simulink model "mds_3c"  (R2014a)
settings: Solver=ode3  StartTime=0.0  StopTime=120  FixedStep=0.002  RelTol=1e-3
settings Model: Creator=john  LastModifiedBy=john

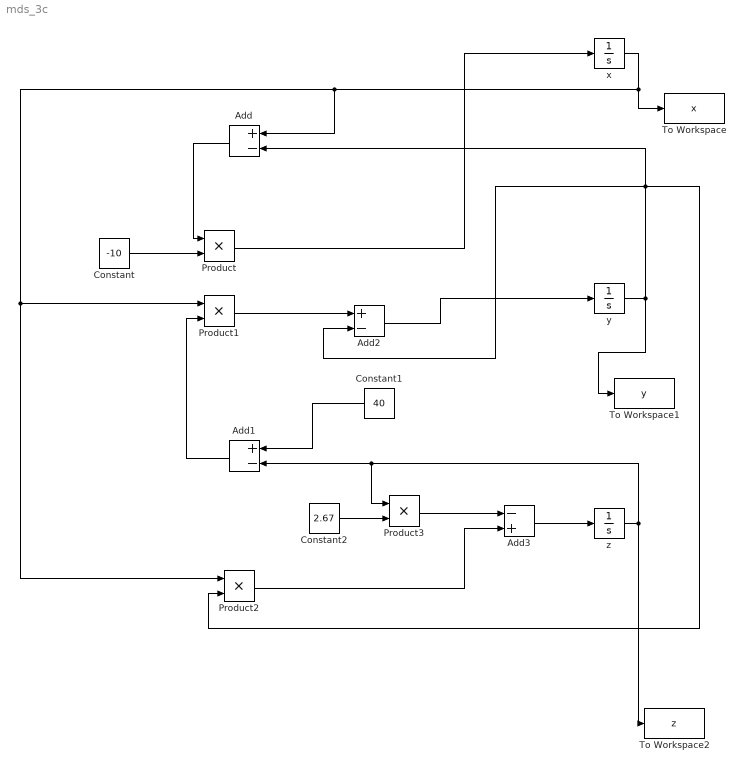
== system mds_3c ==
  Add : Sum  Inputs=+-
  Add1 : Sum  Inputs=+-
  Add2 : Sum  Inputs=+-
  Add3 : Sum  Inputs=-+
  Constant : Constant  Value=-10
  Constant1 : Constant  Value=40
  Constant2 : Constant  Value=2.67
  Product{,1..3} (4 alike) : Product
  To Workspace : ToWorkspace  VariableName=x  SampleTime=-1
  To Workspace1 : ToWorkspace  VariableName=y  SampleTime=-1
  To Workspace2 : ToWorkspace  VariableName=z  SampleTime=-1
  x : Integrator  InitialCondition=0.01
  y : Integrator  InitialCondition=0.01
  z : Integrator
  wires:
  x/1 -> To Workspace/1, Product2/1, Product1/1, Add/1
  Add/1 -> Product/1
  y/1 -> Product2/2, Add/2, Add2/2, To Workspace1/1
  Constant/1 -> Product/2
  z/1 -> Add1/2, Product3/1, To Workspace2/1
  Constant1/1 -> Add1/1
  Add1/1 -> Product1/2
  Product/1 -> x/1
  Product1/1 -> Add2/1
  Add2/1 -> y/1
  Constant2/1 -> Product3/2
  Add3/1 -> z/1
  Product2/1 -> Add3/2
  Product3/1 -> Add3/1
